simulink subsystem "LowLevelController"  (R2023a)
settings: Solver=VariableStepAuto  StartTime=0.0  StopTime=10.0  RelTol=1e-3
model mask{Km=0.3, KLowMkvar=1}
  mask prompts: Km "Momentum motor coeff"; KLowMkvar "Error gain coeff"
settings Model: Creator=user  LastModifiedBy=User

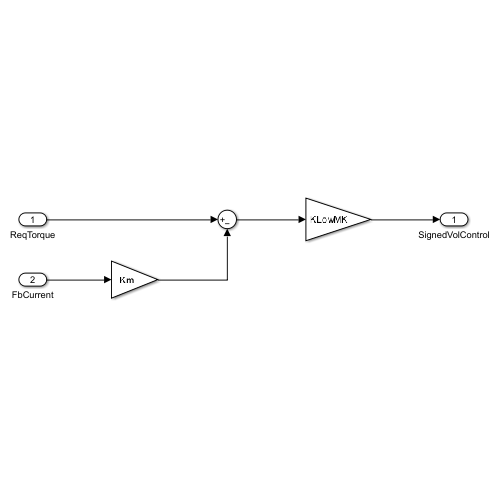
[thumbnail: Simulink's stored preview of the top-level diagram]
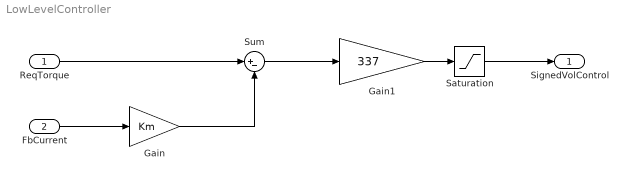
== system LowLevelController ==
  ReqTorque : Inport
  FbCurrent : Inport  Port=2
  Gain : Gain  Gain=Km
  Gain1 : Gain  Gain=337
  Saturation : Saturate  UpperLimit=3.3  LowerLimit=-3.3
  Sum : Sum  Inputs=|+-
  SignedVolControl : Outport
  wires:
  FbCurrent/1 -> Gain/1
  ReqTorque/1 -> Sum/1
  Gain/1 -> Sum/2
  Sum/1 -> Gain1/1
  Gain1/1 -> Saturation/1
  Saturation/1 -> SignedVolControl/1
